simulink model "ipmsm_electrical_test"  (R2015a)
settings: Solver=ode45  StartTime=0.0  StopTime=0.3  RelTol=1e-3
settings Model: Creator=user  LastModifiedBy=user

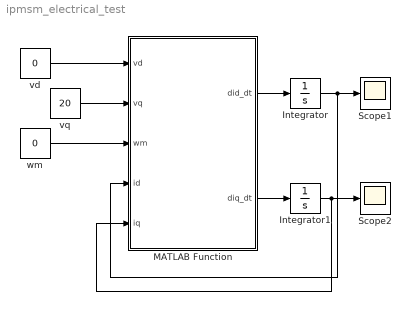
== system ipmsm_electrical_test ==
  Integrator : Integrator
  Integrator1 : Integrator
  MATLAB Function : MATLAB Function  TreatAsAtomicUnit=on
  Scope1 : Scope
  Scope2 : Scope
  vd : Constant  Value=0
  vq : Constant  Value=20
  wm : Constant  Value=0
  wires:
  vd/1 -> MATLAB Function/1(vd)
  vq/1 -> MATLAB Function/2(vq)
  wm/1 -> MATLAB Function/3(wm)
  MATLAB Function/1(did_dt) -> Integrator/1
  Integrator/1 -> Scope1/1, MATLAB Function/4(id)
  MATLAB Function/2(diq_dt) -> Integrator1/1
  Integrator1/1 -> MATLAB Function/5(iq), Scope2/1

== matlab function ipmsm_electrical_test/MATLAB Function ==
  data: vd input; did_dt output; vq input; wm input; id input; iq input; diq_dt output
function [did_dt, diq_dt] = ipmsm_electrical(vd, vq, wm, id, iq)
% BMW i3 IPMSM dq-axis electrical dynamics
% Units: V, rad/s, A, A/s

Rs       = 5.3e-3;    % Stator resistance, Ohm
Ld       = 0.090e-3;  % d-axis inductance, H
Lq       = 0.255e-3;  % q-axis inductance, H
lambda_m = 0.0385;    % PM flux linkage, Wb
p        = 6;         % Pole pairs

we = p*wm;             % electrical angular velocity, rad/s

did_dt = (vd - Rs*id + we*Lq*iq) / Ld;
diq_dt = (vq - Rs*iq - we*(Ld*id + lambda_m)) / Lq;

end
